simulink model "Sensor_Model"  (R2024b)
settings: Solver=VariableStepAuto  StartTime=0.0  StopTime=0.25  RelTol=1e-3
libraries: simulink x6
settings Model: Creator=Zohaib  LastModifiedBy=Zohaib
settings DataIOCC: ReturnWorkspaceOutputs=off

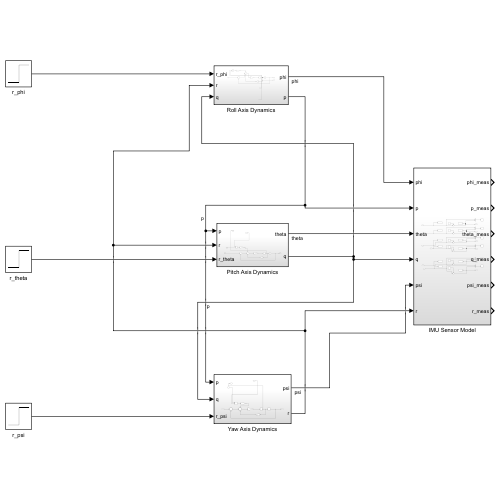
[thumbnail: Simulink's stored preview of the top-level diagram]
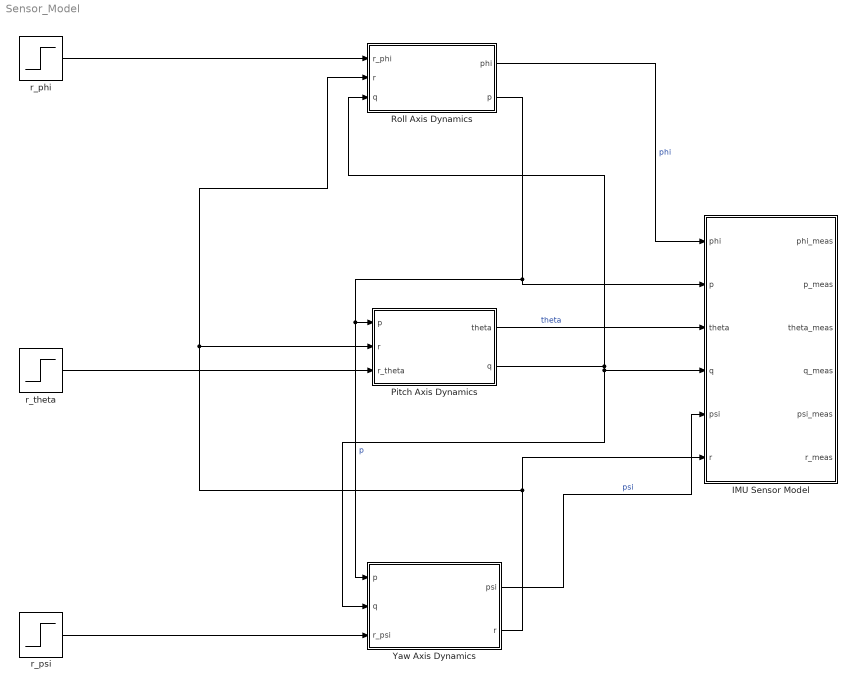
== system Sensor_Model ==
  IMU Sensor Model : Subsystem
  Pitch Axis Dynamics : Subsystem
  Roll Axis Dynamics : Subsystem
  Yaw Axis Dynamics : Subsystem
  r_phi : Step  Time=0  After=1.0001  SampleTime=0
  r_psi : Step  Time=0  After=1.0001  SampleTime=0
  r_theta : Step  Time=0  After=1.0001  SampleTime=0
  wires:
  Roll Axis Dynamics/2(p) -> Yaw Axis Dynamics/1(p), Pitch Axis Dynamics/1(p), IMU Sensor Model/2(p)  "p"
  r_psi/1 -> Yaw Axis Dynamics/3(r_psi)
  r_phi/1 -> Roll Axis Dynamics/1(r_phi)
  r_theta/1 -> Pitch Axis Dynamics/3(r_theta)
  Pitch Axis Dynamics/2(q) -> Yaw Axis Dynamics/2(q), IMU Sensor Model/4(q), Roll Axis Dynamics/3(q)
  Yaw Axis Dynamics/2(r) -> Roll Axis Dynamics/2(r), Pitch Axis Dynamics/2(r), IMU Sensor Model/6(r)
  Roll Axis Dynamics/1(phi) -> IMU Sensor Model/1(phi)  "phi"
  Pitch Axis Dynamics/1(theta) -> IMU Sensor Model/3(theta)  "theta"
  Yaw Axis Dynamics/1(psi) -> IMU Sensor Model/5(psi)  "psi"

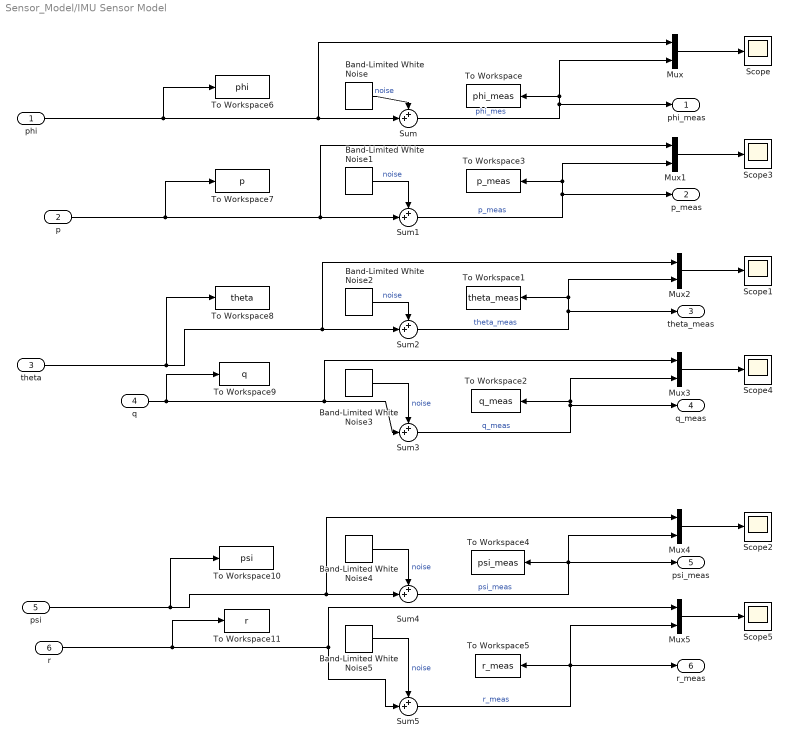
== system Sensor_Model/IMU Sensor Model ==
  phi : Inport
  p : Inport  Port=2
  theta : Inport  Port=3
  q : Inport  Port=4
  psi : Inport  Port=5
  r : Inport  Port=6
  Band-Limited White Noise : simulink/Sources/Band-Limited White Noise  Cov=7.16e-7  Ts=0.001  seed=1
  Band-Limited White Noise1 : simulink/Sources/Band-Limited White Noise  Cov=1.69e-6  Ts=0.001  seed=4
  Band-Limited White Noise2 : simulink/Sources/Band-Limited White Noise  Cov=7.16e-7  Ts=0.001  seed=2
  Band-Limited White Noise3 : simulink/Sources/Band-Limited White Noise  Cov=1.69e-6  Ts=0.001  seed=5
  Band-Limited White Noise4 : simulink/Sources/Band-Limited White Noise  Cov=7.16e-7  Ts=0.001  seed=3
  Band-Limited White Noise5 : simulink/Sources/Band-Limited White Noise  Cov=1.69e-6  Ts=0.001  seed=6
  Mux{,1..5} (6 alike) : Mux  Inputs=2
  Scope{,1..5} (6 alike) : Scope
  Sum{,1..5} (6 alike) : Sum  Inputs=++|
  To Workspace : ToWorkspace  VariableName=phi_meas  SaveFormat=Timeseries  SampleTime=-1
  To Workspace1 : ToWorkspace  VariableName=theta_meas  SaveFormat=Timeseries  SampleTime=-1
  To Workspace10 : ToWorkspace  VariableName=psi  SaveFormat=Timeseries  SampleTime=-1
  To Workspace11 : ToWorkspace  VariableName=r  SaveFormat=Timeseries  SampleTime=-1
  To Workspace2 : ToWorkspace  VariableName=q_meas  SaveFormat=Timeseries  SampleTime=-1
  To Workspace3 : ToWorkspace  VariableName=p_meas  SaveFormat=Timeseries  SampleTime=-1
  To Workspace4 : ToWorkspace  VariableName=psi_meas  SaveFormat=Timeseries  SampleTime=-1
  To Workspace5 : ToWorkspace  VariableName=r_meas  SaveFormat=Timeseries  SampleTime=-1
  To Workspace6 : ToWorkspace  VariableName=phi  SaveFormat=Timeseries  SampleTime=-1
  To Workspace7 : ToWorkspace  VariableName=p  SaveFormat=Timeseries  SampleTime=-1
  To Workspace8 : ToWorkspace  VariableName=theta  SaveFormat=Timeseries  SampleTime=-1
  To Workspace9 : ToWorkspace  VariableName=q  SaveFormat=Timeseries  SampleTime=-1
  phi_meas : Outport
  p_meas : Outport  Port=2
  theta_meas : Outport  Port=3
  q_meas : Outport  Port=4
  psi_meas : Outport  Port=5
  r_meas : Outport  Port=6
  wires:
  Band-Limited White Noise1/1 -> Sum1/1  "noise"
  Band-Limited White Noise3/1 -> Sum3/1  "noise"
  Sum3/1 -> q_meas/1, Mux3/2, To Workspace2/1  "q_meas"
  Sum2/1 -> theta_meas/1, Mux2/2, To Workspace1/1  "theta_meas"
  psi/1 -> To Workspace10/1, Mux4/1, Sum4/2
  Band-Limited White Noise4/1 -> Sum4/1  "noise"
  phi/1 -> To Workspace6/1, Sum/2, Mux/1
  Sum4/1 -> psi_meas/1, Mux4/2, To Workspace4/1  "psi_meas"
  Band-Limited White Noise2/1 -> Sum2/1  "noise"
  q/1 -> To Workspace9/1, Mux3/1, Sum3/2
  Mux/1 -> Scope/1
  Sum1/1 -> p_meas/1, Mux1/2, To Workspace3/1  "p_meas"
  p/1 -> To Workspace7/1, Sum1/2, Mux1/1
  Band-Limited White Noise/1 -> Sum/1  "noise"
  Sum/1 -> phi_meas/1, To Workspace/1, Mux/2  "phi_mes"
  Mux2/1 -> Scope1/1
  Sum5/1 -> To Workspace5/1, r_meas/1, Mux5/2  "r_meas"
  Band-Limited White Noise5/1 -> Sum5/1  "noise"
  Mux3/1 -> Scope4/1
  Mux1/1 -> Scope3/1
  Mux4/1 -> Scope2/1
  theta/1 -> To Workspace8/1, Mux2/1, Sum2/2
  Mux5/1 -> Scope5/1
  r/1 -> To Workspace11/1, Sum5/2, Mux5/1

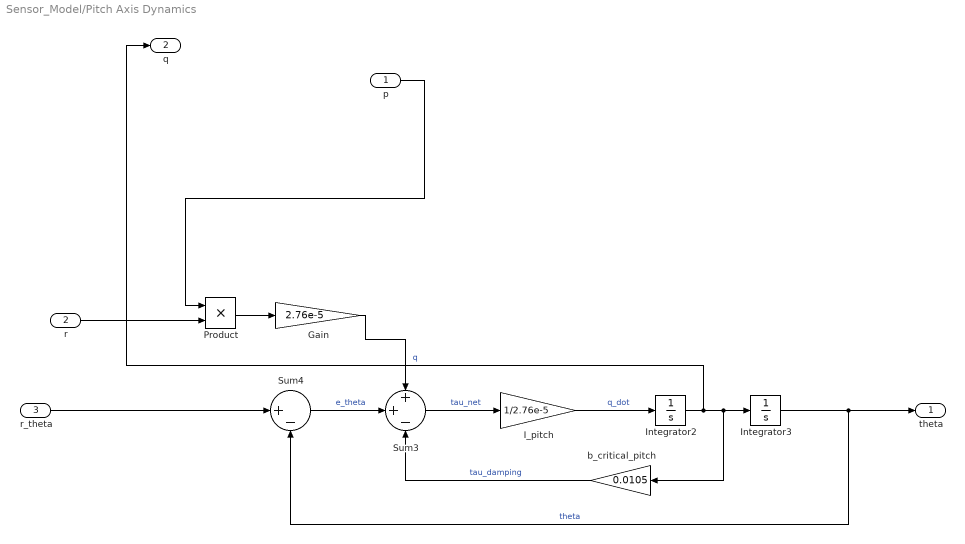
== system Sensor_Model/Pitch Axis Dynamics ==
  p : Inport
  r : Inport  Port=2
  r_theta : Inport  Port=3
  Gain : Gain  Gain=2.76e-5
  I_pitch : Gain  Gain=1/2.76e-5
  Integrator2 : Integrator
  Integrator3 : Integrator
  Product : Product
  Sum3 : Sum  Inputs=++-
  Sum4 : Sum  Inputs=|+-
  b_critical_pitch : Gain  Gain=0.0105
  theta : Outport
  q : Outport  Port=2
  wires:
  r/1 -> Product/2
  Integrator2/1 -> q/1, b_critical_pitch/1, Integrator3/1  "q"
  b_critical_pitch/1 -> Sum3/3  "tau_damping"
  Sum3/1 -> I_pitch/1  "tau_net"
  Product/1 -> Gain/1
  Sum4/1 -> Sum3/2  "e_theta"
  Gain/1 -> Sum3/1
  I_pitch/1 -> Integrator2/1  "q_dot"
  Integrator3/1 -> theta/1, Sum4/2  "theta"
  p/1 -> Product/1
  r_theta/1 -> Sum4/1

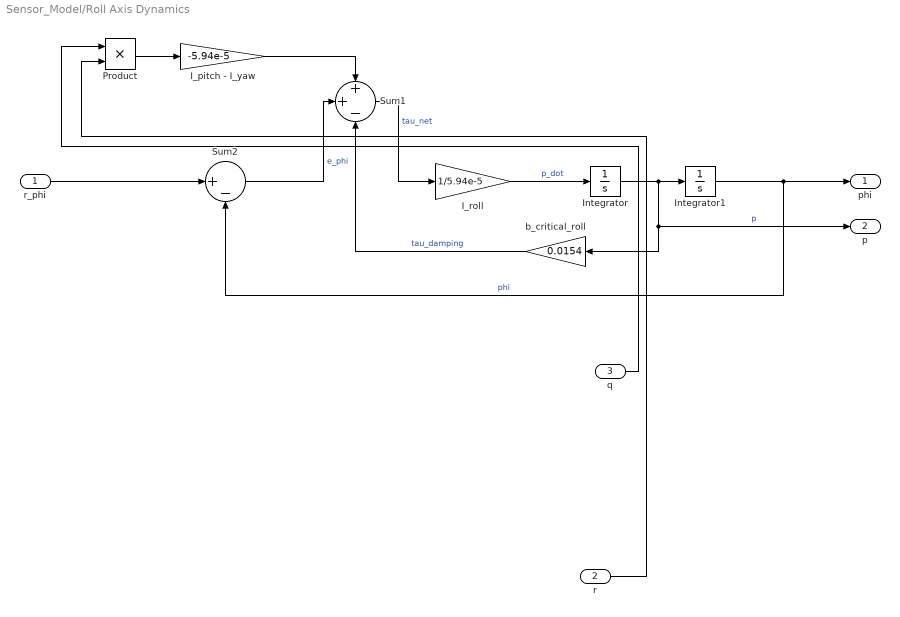
== system Sensor_Model/Roll Axis Dynamics ==
  r_phi : Inport
  r : Inport  Port=2
  q : Inport  Port=3
  I_pitch - I_yaw : Gain  Gain=-5.94e-5
  I_roll : Gain  Gain=1/5.94e-5
  Integrator : Integrator
  Integrator1 : Integrator
  Product : Product
  Sum1 : Sum  Inputs=++-
  Sum2 : Sum  Inputs=|+-
  b_critical_roll : Gain  Gain=0.0154
  phi : Outport
  p : Outport  Port=2
  wires:
  I_pitch - I_yaw/1 -> Sum1/1
  b_critical_roll/1 -> Sum1/3  "tau_damping"
  Integrator1/1 -> phi/1, Sum2/2  "phi"
  Sum2/1 -> Sum1/2  "e_phi"
  Product/1 -> I_pitch - I_yaw/1
  I_roll/1 -> Integrator/1  "p_dot"
  Integrator/1 -> p/1, b_critical_roll/1, Integrator1/1  "p"
  Sum1/1 -> I_roll/1  "tau_net"
  r/1 -> Product/2
  q/1 -> Product/1
  r_phi/1 -> Sum2/1

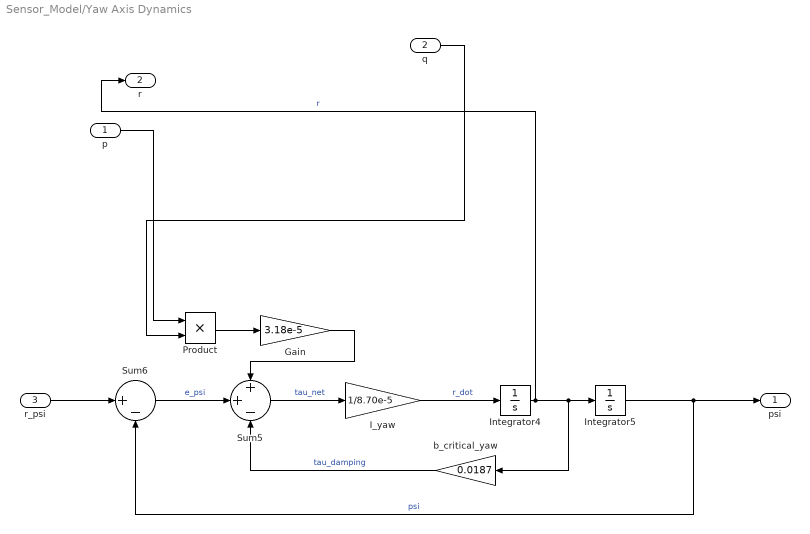
== system Sensor_Model/Yaw Axis Dynamics ==
  p : Inport
  q : Inport  Port=2
  r_psi : Inport  Port=3
  Gain : Gain  Gain=3.18e-5
  I_yaw : Gain  Gain=1/8.70e-5
  Integrator4 : Integrator
  Integrator5 : Integrator
  Product : Product
  Sum5 : Sum  Inputs=++-
  Sum6 : Sum  Inputs=|+-
  b_critical_yaw : Gain  Gain=0.0187
  psi : Outport
  r : Outport  Port=2
  wires:
  Sum6/1 -> Sum5/2  "e_psi"
  Gain/1 -> Sum5/1
  Integrator5/1 -> psi/1, Sum6/2  "psi"
  I_yaw/1 -> Integrator4/1  "r_dot"
  Integrator4/1 -> r/1, b_critical_yaw/1, Integrator5/1  "r"
  q/1 -> Product/2
  b_critical_yaw/1 -> Sum5/3  "tau_damping"
  Product/1 -> Gain/1
  r_psi/1 -> Sum6/1
  p/1 -> Product/1
  Sum5/1 -> I_yaw/1  "tau_net"
